simulink model "controller_pid_sim_noise"  (R2014b)
settings: Solver=ode45  StartTime=0.0  StopTime=10.0  RelTol=1e-3
values from neighbouring files (symbols this model uses):
  g = 9.81    [gain_tuning.m]    (also in gain_tuning_noise.m; model_exp_comparison.m; transfer_functions.m)
  gains = readGains('current_gains.txt')    [gain_tuning_noise.m]    (also in transfer_functions.m)
  noise_phi_mean = 0    [gain_tuning_noise.m]
  noise_theta_mean = 0    [gain_tuning_noise.m]
  vx_sat_max = 1    [gain_tuning.m]    (also in gain_tuning_noise.m = 0.5; model_exp_comparison.m = 0.2)
  vx_sat_min = -1    [gain_tuning.m]    (also in gain_tuning_noise.m = -0.5; model_exp_comparison.m = -0.2)
  vy_sat_max = 1    [gain_tuning.m]    (also in gain_tuning_noise.m = 0.5; model_exp_comparison.m = 0.2)
  vy_sat_min = -1    [gain_tuning.m]    (also in gain_tuning_noise.m = -0.5; model_exp_comparison.m = -0.2)
libraries: simulink x7, commnoisgen2 x2
settings Model: Creator=MARK  LastModifiedBy=MARK

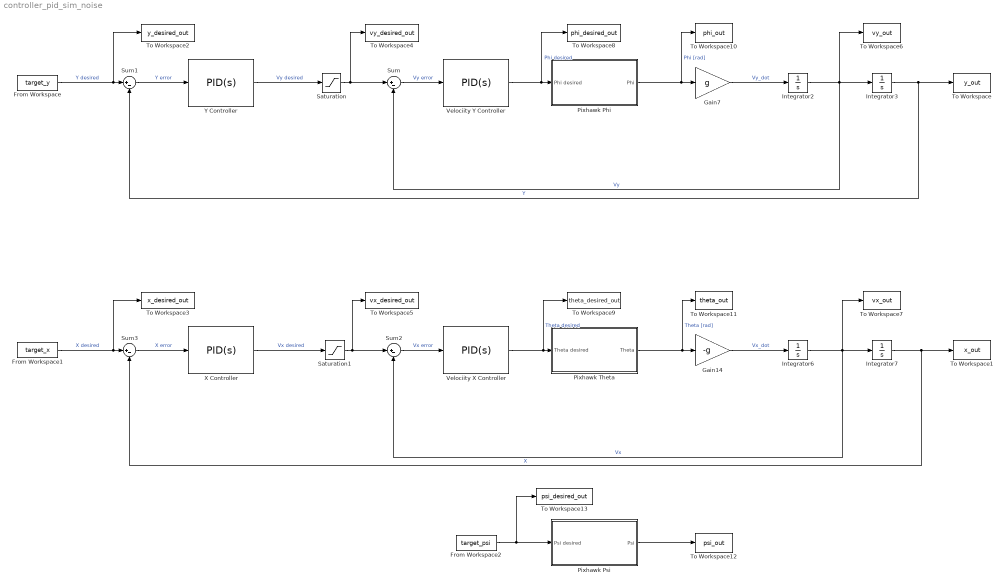
== system controller_pid_sim_noise ==
  From Workspace : FromWorkspace  VariableName=target_y  SampleTime=0
  From Workspace1 : FromWorkspace  VariableName=target_x  SampleTime=0
  From Workspace2 : FromWorkspace  VariableName=target_psi  SampleTime=0
  Gain14 : Gain  Gain=-g
  Gain7 : Gain  Gain=g
  Integrator{2..3,6..7} (4 alike) : Integrator
  Pixhawk Phi : Subsystem
  Pixhawk Psi : Subsystem
  Pixhawk Theta : Subsystem
  Saturation : Saturate  UpperLimit=vx_sat_max  LowerLimit=vx_sat_min
  Saturation1 : Saturate  UpperLimit=vy_sat_max  LowerLimit=vy_sat_min
  Sum{,1..3} (4 alike) : Sum  Inputs=|+-
  To Workspace : ToWorkspace  VariableName=y_out  SaveFormat=Structure With Time  SampleTime=-1
  To Workspace1 : ToWorkspace  VariableName=x_out  SaveFormat=Structure With Time  SampleTime=-1
  To Workspace10 : ToWorkspace  VariableName=phi_out  SaveFormat=Structure With Time  SampleTime=-1
  To Workspace11 : ToWorkspace  VariableName=theta_out  SaveFormat=Structure With Time  SampleTime=-1
  To Workspace12 : ToWorkspace  VariableName=psi_out  SaveFormat=Structure With Time  SampleTime=-1
  To Workspace13 : ToWorkspace  VariableName=psi_desired_out  SaveFormat=Structure With Time  SampleTime=-1
  To Workspace2 : ToWorkspace  VariableName=y_desired_out  SaveFormat=Structure With Time  SampleTime=-1
  To Workspace3 : ToWorkspace  VariableName=x_desired_out  SaveFormat=Structure With Time  SampleTime=-1
  To Workspace4 : ToWorkspace  VariableName=vy_desired_out  SaveFormat=Structure With Time  SampleTime=-1
  To Workspace5 : ToWorkspace  VariableName=vx_desired_out  SaveFormat=Structure With Time  SampleTime=-1
  To Workspace6 : ToWorkspace  VariableName=vy_out  SaveFormat=Structure With Time  SampleTime=-1
  To Workspace7 : ToWorkspace  VariableName=vx_out  SaveFormat=Structure With Time  SampleTime=-1
  To Workspace8 : ToWorkspace  VariableName=phi_desired_out  SaveFormat=Structure With Time  SampleTime=-1
  To Workspace9 : ToWorkspace  VariableName=theta_desired_out  SaveFormat=Structure With Time  SampleTime=-1
  Velociity X Controller : simulink/Continuous/PID Controller  Controller=PID  TimeDomain=Continuous-time  SampleTime=-1  IntegratorMethod=Forward Euler  FilterMethod=Forward Euler  Form=Parallel  P=gains.Pvx  I=gains.Ivx  D=gains.Dvx  N=100  InitialConditionSource=internal  InitialConditionForIntegrator=0  InitialConditionForFilter=0  ExternalReset=none  LimitOutput=off  UpperSaturationLimit=inf  LowerSaturationLimit=-inf  LinearizeAsGain=on  AntiWindupMode=none  Kb=1  TrackingMode=off  Kt=1  PParamMin=[]  PParamMax=[]  IParamMin=[]  IParamMax=[]  DParamMin=[]  DParamMax=[]  NParamMin=[]  NParamMax=[]  KbParamMin=[]  KbParamMax=[]  KtParamMin=[]  KtParamMax=[]  POutMin=[]  POutMax=[]  IOutMin=[]  IOutMax=[]  DOutMin=[]  DOutMax=[]  NOutMin=[]  NOutMax=[]  KbOutMin=[]  KbOutMax=[]  KtOutMin=[]  KtOutMax=[]  IntegratorOutMin=[]  IntegratorOutMax=[]  FilterOutMin=[]  FilterOutMax=[]  SumOutMin=[]  SumOutMax=[]  SumI1OutMin=[]  SumI1OutMax=[]  SumI2OutMin=[]  SumI2OutMax=[]  SumI3OutMin=[]  SumI3OutMax=[]  SumDOutMin=[]  SumDOutMax=[]  SaturationOutMin=[]  SaturationOutMax=[]  IntegratorContinuousStateAttributes=''  IntegratorStateMustResolveToSignalObject=off  IntegratorRTWStateStorageClass=Auto  FilterContinuousStateAttributes=''  FilterStateMustResolveToSignalObject=off  FilterRTWStateStorageClass=Auto  DifferentiatorICPrevScaledInput=0  DifferentiatorOutMin=[]  DifferentiatorOutMax=[]  UseFilter=on
  Velociity Y Controller : simulink/Continuous/PID Controller  Controller=PID  TimeDomain=Continuous-time  SampleTime=-1  IntegratorMethod=Forward Euler  FilterMethod=Forward Euler  Form=Parallel  P=gains.Pvy  I=gains.Ivy  D=gains.Dvy  N=100  InitialConditionSource=internal  InitialConditionForIntegrator=0  InitialConditionForFilter=0  ExternalReset=none  LimitOutput=off  UpperSaturationLimit=inf  LowerSaturationLimit=-inf  LinearizeAsGain=on  AntiWindupMode=none  Kb=1  TrackingMode=off  Kt=1  PParamMin=[]  PParamMax=[]  IParamMin=[]  IParamMax=[]  DParamMin=[]  DParamMax=[]  NParamMin=[]  NParamMax=[]  KbParamMin=[]  KbParamMax=[]  KtParamMin=[]  KtParamMax=[]  POutMin=[]  POutMax=[]  IOutMin=[]  IOutMax=[]  DOutMin=[]  DOutMax=[]  NOutMin=[]  NOutMax=[]  KbOutMin=[]  KbOutMax=[]  KtOutMin=[]  KtOutMax=[]  IntegratorOutMin=[]  IntegratorOutMax=[]  FilterOutMin=[]  FilterOutMax=[]  SumOutMin=[]  SumOutMax=[]  SumI1OutMin=[]  SumI1OutMax=[]  SumI2OutMin=[]  SumI2OutMax=[]  SumI3OutMin=[]  SumI3OutMax=[]  SumDOutMin=[]  SumDOutMax=[]  SaturationOutMin=[]  SaturationOutMax=[]  IntegratorContinuousStateAttributes=''  IntegratorStateMustResolveToSignalObject=off  IntegratorRTWStateStorageClass=Auto  FilterContinuousStateAttributes=''  FilterStateMustResolveToSignalObject=off  FilterRTWStateStorageClass=Auto  DifferentiatorICPrevScaledInput=0  DifferentiatorOutMin=[]  DifferentiatorOutMax=[]  UseFilter=on
  X Controller : simulink/Continuous/PID Controller  Controller=PID  TimeDomain=Continuous-time  SampleTime=-1  IntegratorMethod=Forward Euler  FilterMethod=Forward Euler  Form=Parallel  P=gains.Px  I=gains.Ix  D=gains.Dx  N=100  InitialConditionSource=internal  InitialConditionForIntegrator=0  InitialConditionForFilter=0  ExternalReset=none  LimitOutput=off  UpperSaturationLimit=inf  LowerSaturationLimit=-inf  LinearizeAsGain=on  AntiWindupMode=none  Kb=1  TrackingMode=off  Kt=1  PParamMin=[]  PParamMax=[]  IParamMin=[]  IParamMax=[]  DParamMin=[]  DParamMax=[]  NParamMin=[]  NParamMax=[]  KbParamMin=[]  KbParamMax=[]  KtParamMin=[]  KtParamMax=[]  POutMin=[]  POutMax=[]  IOutMin=[]  IOutMax=[]  DOutMin=[]  DOutMax=[]  NOutMin=[]  NOutMax=[]  KbOutMin=[]  KbOutMax=[]  KtOutMin=[]  KtOutMax=[]  IntegratorOutMin=[]  IntegratorOutMax=[]  FilterOutMin=[]  FilterOutMax=[]  SumOutMin=[]  SumOutMax=[]  SumI1OutMin=[]  SumI1OutMax=[]  SumI2OutMin=[]  SumI2OutMax=[]  SumI3OutMin=[]  SumI3OutMax=[]  SumDOutMin=[]  SumDOutMax=[]  SaturationOutMin=[]  SaturationOutMax=[]  IntegratorContinuousStateAttributes=''  IntegratorStateMustResolveToSignalObject=off  IntegratorRTWStateStorageClass=Auto  FilterContinuousStateAttributes=''  FilterStateMustResolveToSignalObject=off  FilterRTWStateStorageClass=Auto  DifferentiatorICPrevScaledInput=0  DifferentiatorOutMin=[]  DifferentiatorOutMax=[]  UseFilter=on
  Y Controller : simulink/Continuous/PID Controller  Controller=PID  TimeDomain=Continuous-time  SampleTime=-1  IntegratorMethod=Forward Euler  FilterMethod=Forward Euler  Form=Parallel  P=gains.Py  I=gains.Iy  D=gains.Dy  N=100  InitialConditionSource=internal  InitialConditionForIntegrator=0  InitialConditionForFilter=0  ExternalReset=none  LimitOutput=off  UpperSaturationLimit=inf  LowerSaturationLimit=-inf  LinearizeAsGain=on  AntiWindupMode=none  Kb=1  TrackingMode=off  Kt=1  PParamMin=[]  PParamMax=[]  IParamMin=[]  IParamMax=[]  DParamMin=[]  DParamMax=[]  NParamMin=[]  NParamMax=[]  KbParamMin=[]  KbParamMax=[]  KtParamMin=[]  KtParamMax=[]  POutMin=[]  POutMax=[]  IOutMin=[]  IOutMax=[]  DOutMin=[]  DOutMax=[]  NOutMin=[]  NOutMax=[]  KbOutMin=[]  KbOutMax=[]  KtOutMin=[]  KtOutMax=[]  IntegratorOutMin=[]  IntegratorOutMax=[]  FilterOutMin=[]  FilterOutMax=[]  SumOutMin=[]  SumOutMax=[]  SumI1OutMin=[]  SumI1OutMax=[]  SumI2OutMin=[]  SumI2OutMax=[]  SumI3OutMin=[]  SumI3OutMax=[]  SumDOutMin=[]  SumDOutMax=[]  SaturationOutMin=[]  SaturationOutMax=[]  IntegratorContinuousStateAttributes=''  IntegratorStateMustResolveToSignalObject=off  IntegratorRTWStateStorageClass=Auto  FilterContinuousStateAttributes=''  FilterStateMustResolveToSignalObject=off  FilterRTWStateStorageClass=Auto  DifferentiatorICPrevScaledInput=0  DifferentiatorOutMin=[]  DifferentiatorOutMax=[]  UseFilter=on
  wires:
  Pixhawk Phi/1(Phi) -> To Workspace10/1, Gain7/1  "Phi [rad]"
  Gain7/1 -> Integrator2/1  "Vy_dot"
  Integrator2/1 -> To Workspace6/1, Sum/2, Integrator3/1  "Vy"
  Integrator3/1 -> Sum1/2, To Workspace/1  "Y"
  From Workspace/1 -> To Workspace2/1, Sum1/1  "Y desired"
  Gain14/1 -> Integrator6/1  "Vx_dot"
  Integrator6/1 -> To Workspace7/1, Sum2/2, Integrator7/1  "Vx"
  Integrator7/1 -> Sum3/2, To Workspace1/1  "X"
  From Workspace1/1 -> To Workspace3/1, Sum3/1  "X desired"
  Pixhawk Theta/1(Theta) -> To Workspace11/1, Gain14/1  "Theta [rad]"
  Velociity Y Controller/1 -> To Workspace8/1, Pixhawk Phi/1(Phi desired)  "Phi desired"
  Sum/1 -> Velociity Y Controller/1  "Vy error"
  Y Controller/1 -> Saturation/1  "Vy desired"
  Sum1/1 -> Y Controller/1  "Y error"
  Velociity X Controller/1 -> To Workspace9/1, Pixhawk Theta/1(Theta desired)  "Theta desired"
  Sum2/1 -> Velociity X Controller/1  "Vx error"
  X Controller/1 -> Saturation1/1  "Vx desired"
  Sum3/1 -> X Controller/1  "X error"
  Saturation/1 -> To Workspace4/1, Sum/1
  Saturation1/1 -> To Workspace5/1, Sum2/1
  From Workspace2/1 -> To Workspace13/1, Pixhawk Psi/1(Psi desired)
  Pixhawk Psi/1(Psi) -> To Workspace12/1

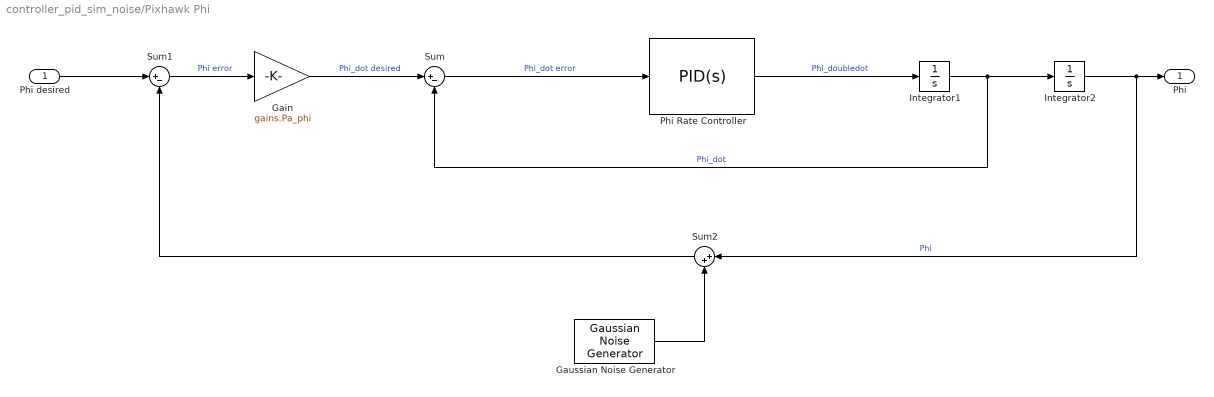
== system controller_pid_sim_noise/Pixhawk Phi ==
  Phi desired : Inport
  Gain : Gain  Gain=gains.Pa_phi
  Gaussian Noise Generator : commnoisgen2/Gaussian Noise Generator  m=noise_phi_mean  d=noise_phi_var  s=41  Ts=1  frameBased=off  sampPerFrame=1  orient=off  outDataType=double
  Integrator1 : Integrator
  Integrator2 : Integrator
  Phi Rate Controller : simulink/Continuous/PID Controller  Controller=PID  TimeDomain=Continuous-time  SampleTime=-1  IntegratorMethod=Forward Euler  FilterMethod=Forward Euler  Form=Parallel  P=gains.Pr_phi  I=gains.Ir_phi  D=gains.Dr_phi  N=100  InitialConditionSource=internal  InitialConditionForIntegrator=0  InitialConditionForFilter=0  ExternalReset=none  LimitOutput=off  UpperSaturationLimit=inf  LowerSaturationLimit=-inf  LinearizeAsGain=on  AntiWindupMode=none  Kb=1  TrackingMode=off  Kt=1  PParamMin=[]  PParamMax=[]  IParamMin=[]  IParamMax=[]  DParamMin=[]  DParamMax=[]  NParamMin=[]  NParamMax=[]  KbParamMin=[]  KbParamMax=[]  KtParamMin=[]  KtParamMax=[]  POutMin=[]  POutMax=[]  IOutMin=[]  IOutMax=[]  DOutMin=[]  DOutMax=[]  NOutMin=[]  NOutMax=[]  KbOutMin=[]  KbOutMax=[]  KtOutMin=[]  KtOutMax=[]  IntegratorOutMin=[]  IntegratorOutMax=[]  FilterOutMin=[]  FilterOutMax=[]  SumOutMin=[]  SumOutMax=[]  SumI1OutMin=[]  SumI1OutMax=[]  SumI2OutMin=[]  SumI2OutMax=[]  SumI3OutMin=[]  SumI3OutMax=[]  SumDOutMin=[]  SumDOutMax=[]  SaturationOutMin=[]  SaturationOutMax=[]  IntegratorContinuousStateAttributes=''  IntegratorStateMustResolveToSignalObject=off  IntegratorRTWStateStorageClass=Auto  FilterContinuousStateAttributes=''  FilterStateMustResolveToSignalObject=off  FilterRTWStateStorageClass=Auto  DifferentiatorICPrevScaledInput=0  DifferentiatorOutMin=[]  DifferentiatorOutMax=[]  UseFilter=on
  Sum : Sum  Inputs=|+-
  Sum1 : Sum  Inputs=|+-
  Sum2 : Sum  Inputs=|++
  Phi : Outport
  wires:
  Integrator2/1 -> Sum2/1, Phi/1  "Phi"
  Integrator1/1 -> Sum/2, Integrator2/1  "Phi_dot"
  Gain/1 -> Sum/1  "Phi_dot desired"
  Phi desired/1 -> Sum1/1
  Sum1/1 -> Gain/1  "Phi error"
  Phi Rate Controller/1 -> Integrator1/1  "Phi_doubledot"
  Sum/1 -> Phi Rate Controller/1  "Phi_dot error"
  Sum2/1 -> Sum1/2
  Gaussian Noise Generator/1 -> Sum2/2

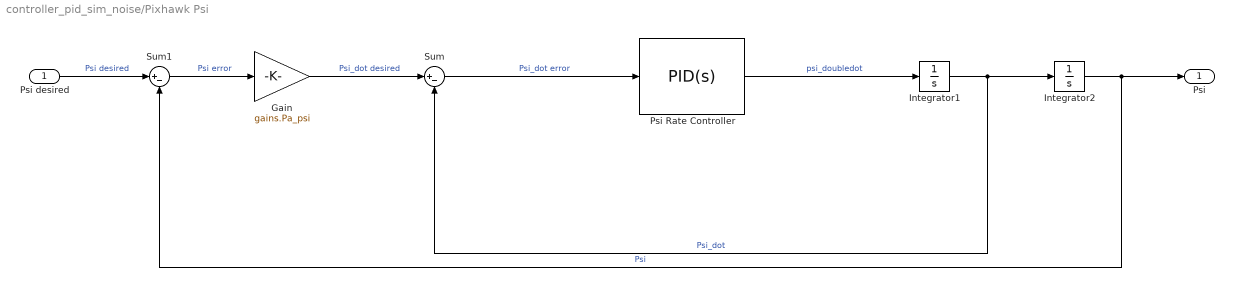
== system controller_pid_sim_noise/Pixhawk Psi ==
  Psi desired : Inport
  Gain : Gain  Gain=gains.Pa_psi
  Integrator1 : Integrator
  Integrator2 : Integrator
  Psi Rate Controller : simulink/Continuous/PID Controller  Controller=PID  TimeDomain=Continuous-time  SampleTime=-1  IntegratorMethod=Forward Euler  FilterMethod=Forward Euler  Form=Parallel  P=gains.Pr_psi  I=gains.Ir_psi  D=gains.Dr_psi  N=100  InitialConditionSource=internal  InitialConditionForIntegrator=0  InitialConditionForFilter=0  ExternalReset=none  LimitOutput=off  UpperSaturationLimit=inf  LowerSaturationLimit=-inf  LinearizeAsGain=on  AntiWindupMode=none  Kb=1  TrackingMode=off  Kt=1  PParamMin=[]  PParamMax=[]  IParamMin=[]  IParamMax=[]  DParamMin=[]  DParamMax=[]  NParamMin=[]  NParamMax=[]  KbParamMin=[]  KbParamMax=[]  KtParamMin=[]  KtParamMax=[]  POutMin=[]  POutMax=[]  IOutMin=[]  IOutMax=[]  DOutMin=[]  DOutMax=[]  NOutMin=[]  NOutMax=[]  KbOutMin=[]  KbOutMax=[]  KtOutMin=[]  KtOutMax=[]  IntegratorOutMin=[]  IntegratorOutMax=[]  FilterOutMin=[]  FilterOutMax=[]  SumOutMin=[]  SumOutMax=[]  SumI1OutMin=[]  SumI1OutMax=[]  SumI2OutMin=[]  SumI2OutMax=[]  SumI3OutMin=[]  SumI3OutMax=[]  SumDOutMin=[]  SumDOutMax=[]  SaturationOutMin=[]  SaturationOutMax=[]  IntegratorContinuousStateAttributes=''  IntegratorStateMustResolveToSignalObject=off  IntegratorRTWStateStorageClass=Auto  FilterContinuousStateAttributes=''  FilterStateMustResolveToSignalObject=off  FilterRTWStateStorageClass=Auto  DifferentiatorICPrevScaledInput=0  DifferentiatorOutMin=[]  DifferentiatorOutMax=[]  UseFilter=on
  Sum : Sum  Inputs=|+-
  Sum1 : Sum  Inputs=|+-
  Psi : Outport
  wires:
  Integrator2/1 -> Psi/1, Sum1/2  "Psi"
  Integrator1/1 -> Sum/2, Integrator2/1  "Psi_dot"
  Gain/1 -> Sum/1  "Psi_dot desired"
  Psi desired/1 -> Sum1/1  "Psi desired"
  Sum1/1 -> Gain/1  "Psi error"
  Psi Rate Controller/1 -> Integrator1/1  "psi_doubledot"
  Sum/1 -> Psi Rate Controller/1  "Psi_dot error"

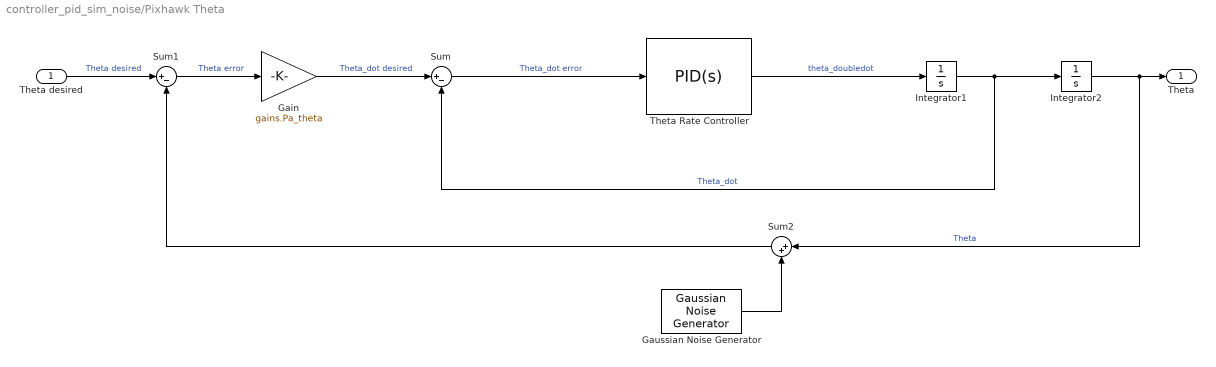
== system controller_pid_sim_noise/Pixhawk Theta ==
  Theta desired : Inport
  Gain : Gain  Gain=gains.Pa_theta
  Gaussian Noise Generator : commnoisgen2/Gaussian Noise Generator  m=noise_theta_mean  d=noise_theta_var  s=41  Ts=1  frameBased=off  sampPerFrame=1  orient=off  outDataType=double
  Integrator1 : Integrator
  Integrator2 : Integrator
  Sum : Sum  Inputs=|+-
  Sum1 : Sum  Inputs=|+-
  Sum2 : Sum  Inputs=|++
  Theta Rate Controller : simulink/Continuous/PID Controller  Controller=PID  TimeDomain=Continuous-time  SampleTime=-1  IntegratorMethod=Forward Euler  FilterMethod=Forward Euler  Form=Parallel  P=gains.Pr_theta  I=gains.Ir_theta  D=gains.Dr_theta  N=100  InitialConditionSource=internal  InitialConditionForIntegrator=0  InitialConditionForFilter=0  ExternalReset=none  LimitOutput=off  UpperSaturationLimit=inf  LowerSaturationLimit=-inf  LinearizeAsGain=on  AntiWindupMode=none  Kb=1  TrackingMode=off  Kt=1  PParamMin=[]  PParamMax=[]  IParamMin=[]  IParamMax=[]  DParamMin=[]  DParamMax=[]  NParamMin=[]  NParamMax=[]  KbParamMin=[]  KbParamMax=[]  KtParamMin=[]  KtParamMax=[]  POutMin=[]  POutMax=[]  IOutMin=[]  IOutMax=[]  DOutMin=[]  DOutMax=[]  NOutMin=[]  NOutMax=[]  KbOutMin=[]  KbOutMax=[]  KtOutMin=[]  KtOutMax=[]  IntegratorOutMin=[]  IntegratorOutMax=[]  FilterOutMin=[]  FilterOutMax=[]  SumOutMin=[]  SumOutMax=[]  SumI1OutMin=[]  SumI1OutMax=[]  SumI2OutMin=[]  SumI2OutMax=[]  SumI3OutMin=[]  SumI3OutMax=[]  SumDOutMin=[]  SumDOutMax=[]  SaturationOutMin=[]  SaturationOutMax=[]  IntegratorContinuousStateAttributes=''  IntegratorStateMustResolveToSignalObject=off  IntegratorRTWStateStorageClass=Auto  FilterContinuousStateAttributes=''  FilterStateMustResolveToSignalObject=off  FilterRTWStateStorageClass=Auto  DifferentiatorICPrevScaledInput=0  DifferentiatorOutMin=[]  DifferentiatorOutMax=[]  UseFilter=on
  Theta : Outport
  wires:
  Integrator2/1 -> Sum2/1, Theta/1  "Theta"
  Integrator1/1 -> Sum/2, Integrator2/1  "Theta_dot"
  Gain/1 -> Sum/1  "Theta_dot desired"
  Theta desired/1 -> Sum1/1  "Theta desired"
  Sum1/1 -> Gain/1  "Theta error"
  Theta Rate Controller/1 -> Integrator1/1  "theta_doubledot"
  Sum/1 -> Theta Rate Controller/1  "Theta_dot error"
  Sum2/1 -> Sum1/2
  Gaussian Noise Generator/1 -> Sum2/2
